simulink model "GhendyanoT2F"  (R2021b)
settings: Solver=ode45  StartTime=0.0  StopTime=TempoSimulacao  RelTol=1e-3  EnableMultiTasking=on
values from neighbouring files (symbols this model uses):
  ccc1 = Ccc*d    [TesteRealCurtoFuses.m]    (also in TesteRealCurto_SemFuse.m)
  ccc2 = Ccc*d    [TesteRealCurtoFuses.m]    (also in TesteRealCurto_SemFuse.m)
  cct1 = Cct*d    [TesteRealCurtoFuses.m]    (also in TesteRealCurto_SemFuse.m)
  cct2 = Cct*d    [TesteRealCurtoFuses.m]    (also in TesteRealCurto_SemFuse.m)
  cequa1 = Ceq*d    [TesteRealCurtoFuses.m]    (also in TesteRealCurto_SemFuse.m)
  cequa2 = Ceq*d    [TesteRealCurtoFuses.m]    (also in TesteRealCurto_SemFuse.m)
  FatorSimulacao = 1e-3    (= 0.001)    [TesteRealCurtoFuses.m]    (also in TesteRealCurto_SemFuse.m)
  le = 1e-10    [TesteRealCurto.m]    (also in TesteRealCurtoFuses.m; TesteRealCurto_SemFuse.m)
  lm1 = lm    [TesteRealCurto.m]    (also in TesteRealCurtoFuses.m; TesteRealCurto_SemFuse.m)
  lm2 = lm    [TesteRealCurto.m]    (also in TesteRealCurtoFuses.m; TesteRealCurto_SemFuse.m)
  lp1 = lp    [TesteRealCurto.m]    (also in TesteRealCurtoFuses.m; TesteRealCurto_SemFuse.m)
  lp2 = lp    [TesteRealCurto.m]    (also in TesteRealCurtoFuses.m; TesteRealCurto_SemFuse.m)
  NRE = 1e-12    [TesteRealCurto.m]    (also in TesteRealCurtoFuses.m; TesteRealCurto_SemFuse.m)
  Raf1 = inf    [TesteRealCurto.m]    (also in TesteRealCurtoFuses.m; TesteRealCurto_SemFuse.m)
  Raf2 = inf    [TesteRealCurto.m]    (also in TesteRealCurtoFuses.m; TesteRealCurto_SemFuse.m)
  Rbf1 = inf    [TesteRealCurto.m]    (also in TesteRealCurtoFuses.m; TesteRealCurto_SemFuse.m)
  Rbf2 = inf    [TesteRealCurto.m]    (also in TesteRealCurtoFuses.m; TesteRealCurto_SemFuse.m)
  Rcf1 = inf    [TesteRealCurto.m]    (also in TesteRealCurtoFuses.m; TesteRealCurto_SemFuse.m)
  Rcf2 = inf    [TesteRealCurto.m]    (also in TesteRealCurtoFuses.m; TesteRealCurto_SemFuse.m)
  rm1 = rm    [TesteRealCurto.m]    (also in TesteRealCurtoFuses.m; TesteRealCurto_SemFuse.m)
  rm2 = rm    [TesteRealCurto.m]    (also in TesteRealCurtoFuses.m; TesteRealCurto_SemFuse.m)
  rp1 = rp    [TesteRealCurto.m]    (also in TesteRealCurtoFuses.m; TesteRealCurto_SemFuse.m)
  rp2 = rp    [TesteRealCurto.m]    (also in TesteRealCurtoFuses.m; TesteRealCurto_SemFuse.m)
  rtc1 = 8    [TesteRealCurto.m]    (also in TesteRealCurtoFuses.m; TesteRealCurto_SemFuse.m)
  rtc2 = 8    [TesteRealCurto.m]    (also in TesteRealCurtoFuses.m; TesteRealCurto_SemFuse.m)
  rti = 10    [TesteRealCurto.m]    (also in TesteRealCurtoFuses.m; TesteRealCurto_SemFuse.m)
undefined symbols (not defined in the file or in its folder): D11, Delta
libraries: spsSeriesRLCBranchLib x26, spsRMSLib x14, spsBreakerLib x9, spsCurrentMeasurementLib x9, spsThreePhaseTransformerTwoWindingsLib x4, spsThreePhaseVIMeasurementLib x3, spsMutualInductanceLib x2, spsThreePhaseSeriesRLCLoadLib x2, spsThreePhaseSourceLib x1, spspowerguiLib x1
(part 1 of 2)
settings Model: Creator=laris  LastModifiedBy=Leonardo-Felipe
settings SolverCC: AlgebraicLoopSolver=TrustRegion
settings DataIOCC: LimitDataPoints=on  SaveFormat=Array  ReturnWorkspaceOutputs=off
settings OptimizationCC: LifeSpan=inf
settings DebuggingCC: SFUnexpectedBacktrackingDiag=warning  SFNoUnconditionalDefaultTransitionDiag=warning  SFExecutionAtInitializationDiag=none  SFMachineParentedDataDiag=warning  ArithmeticOperatorsInVariantConditions=warning
settings HardwareCC: ProdBitPerPointer=32  ProdBitPerSizeT=32  ProdBitPerPtrDiffT=32  ProdLargestAtomicFloat=None  ProdIntDivRoundTo=Undefined  ProdEndianess=Unspecified  ProdWordSize=32  ProdHWDeviceType=32-bit Generic
settings ModelReferenceCC: PropagateSignalLabelsOutOfModel=off
settings SFSimCC: SimUseLocalCustomCode=off  CustomCodeUndefinedFunction=UseInterfaceOnly
settings RTWCC: RTWUseLocalCustomCode=off
settings CodeAppCC: StateflowObjectComments=on
settings GRTTargetCC: TargetLangStandard=C89/C90 (ANSI)
settings ConfigComp: CovMetricSettings=dw  CovSaveCumulativeToWorkspaceVar=on  CovSaveSingleToWorkspaceVar=on  CovExternalEMLEnable=off
settings SimscapeCC: SimscapeNormalizeSystem=off

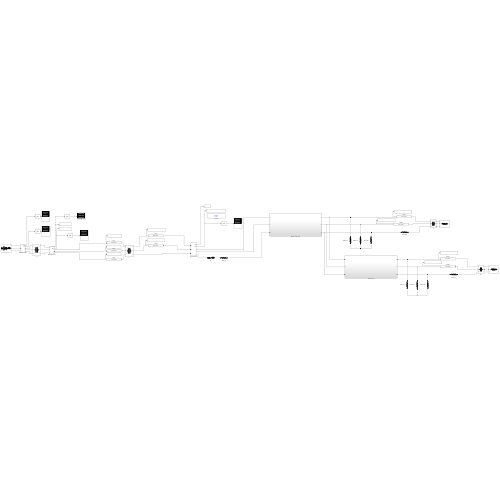
[thumbnail: Simulink's stored preview of the top-level diagram]
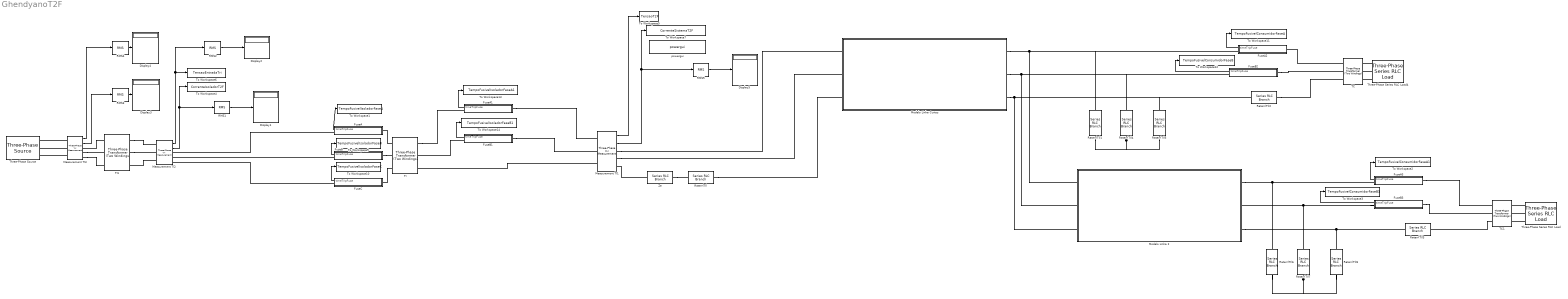
== system GhendyanoT2F ==
  Display{1..5} (5 alike) : Display
  FuseA : Subsystem  mask{tipofuse=5H, a=33.5364, b=-24.1389, c=7.0071, d=-1.0167, e=0.0569, IoTot=5}
      mask prompts: tipofuse "Tipo de Fusivel"
      mask TypeOptions tipofuse: 5H
      mask Callback tipofuse:
      | switch(get_param(gcb,'tipofuse'))
      |     case '1H'
      |         set_param(gcb,'a','11.5834');
      |         set_param(gcb,'b','-7.7159');
      |         set_param(gcb,'c','2.2435');
      |         set_param(gcb,'d','-0.4141');
      |         set_param(gcb,'e','0.0293');
      |         set_param(gcb,'IoTot','1');
      |     case '2H'
      |         set_param(gcb,'a','15.3612');
      |         set_param(gcb,'b','-11.3048');
      |         set_param(gcb,'c','3.7855');
      |         set_param(gcb,'d','-0.6767');
      |         set_param(gcb,'e','0.0442');
      |         set_param(gcb,'IoTot','2');
      |     case '3H'
      |         set_param(gcb,'a','16.6469');
      |         set_param(gcb,'b','-10.3608');
      |         set_param(gcb,'c','2.8987');
      |         set_param(gcb,'d','-0.4844');
      |         set_param(gcb,'e','0.0315');
      |         set_param(gcb,'IoTot','3');
      |     case '5H'
      |         set_param(gcb,'a','33.5364');
      |         set_param(gcb,'b','-24.1389');
      |         set_param(gcb,'c','7.0071');
      |         set_param(gcb,'d','-1.0167');
      |         set_param(gcb,'e','0.0569');
      |         set_param(gcb,'IoTot','5');
      |     case '8H'
      |         set_param(gcb,'a','137.5572');
      |         set_param(gcb,'b','-119.0117');
      |         set_param(gcb,'c','38.2794');
      |         set_param(gcb,'d','-5.4440');
      |         set_param(gcb,'e','0.2846');
      |         set_param(gcb,'IoTot','8');
      |     case '6K'
      |         set_param(gcb,'a','181.2568');
      |         set_param(gcb,'b','-167.5711');
      |         set_param(gcb,'c','57.6673');
      |         set_param(gcb,'d','-8.7672');
      |         set_param(gcb,'e','0.4916');
      |         set_param(gcb,'IoTot','6');
      |     case '8K'
      |         set_param(gcb,'a','201.6778');
      |         set_param(gcb,'b','-175.2376');
      |         set_param(gcb,'c','56.8760');
      |         set_param(gcb,'d','-8.1725');
      |         set_param(gcb,'e','0.4340');
      |         set_param(gcb,'IoTot','8');
      |     case '10K'
      |         set_param(gcb,'a','251.8801');
      |         set_param(gcb,'b','-206.6378');
      |         set_param(gcb,'c','63.3069');
      |         set_param(gcb,'d','-8.5810');
      |         set_param(gcb,'e','0.4304');
      |         set_param(gcb,'IoTot','10');
      |     case '12K'
      |         set_param(gcb,'a','294.2461');
      |         set_param(gcb,'b','-229.0340');
      |         set_param(gcb,'c','66.6693');
      |         set_param(gcb,'d','-8.5945');
      |         set_param(gcb,'e','0.4107');
      |         set_param(gcb,'IoTot','12');
      |     case '15K'
      |         set_param(gcb,'a','346.4070');
      |         set_param(gcb,'b','-257.6697');
      |         set_param(gcb,'c','71.6644');
      |         set_param(gcb,'d','-8.8225');
      |         set_param(gcb,'e','0.4027');
      |         set_param(gcb,'IoTot','15');
      |     case '20K'
      |         set_param(gcb,'a','382.4620');
      |         set_param(gcb,'b','-271.3985');
      |         set_param(gcb,'c','72.1161');
      |         set_param(gcb,'d','-8.4924');
      |         set_param(gcb,'e','0.3714');
      |         set_param(gcb,'IoTot','20');
      |     case '25K'
      |         set_param(gcb,'a','469.9755');
      |         set_param(gcb,'b','-321.2512');
      |         set_param(gcb,'c','82.1749');
      |         set_param(gcb,'d','-9.3092');
      |         set_param(gcb,'e','0.3918');
      |         set_param(gcb,'IoTot','25');
      |     case '30K'
      |         set_param(gcb,'a','516.7220');
      |         set_param(gcb,'b','-337.6034');
      |         set_param(gcb,'c','82.5876');
      |         set_param(gcb,'d','-8.9522');
      |         set_param(gcb,'e','0.3608');
      |         set_param(gcb,'IoTot','30');
      |     case '40K'
      |         set_param(gcb,'a','672.1360');
      |         set_param(gcb,'b','-424.7867');
      |         set_param(gcb,'c','100.3706');
      |         set_param(gcb,'d','-10.4950');
      |         set_param(gcb,'e','0.4080');
      |         set_param(gcb,'IoTot','40');
      |     case '50K'
      |         set_param(gcb,'a','691.3953');
      |         set_param(gcb,'b','-419.2300');
      |         set_param(gcb,'c','95.1730');
      |         set_param(gcb,'d','-9.5735');
      |         set_param(gcb,'e','0.3584');
      |         set_param(gcb,'IoTot','50');
      |     case '65K'
      |         set_param(gcb,'a','841.8993');
      |         set_param(gcb,'b','-492.8148');
      |         set_param(gcb,'c','107.9499');
      |         set_param(gcb,'d','-10.4731');
      |         set_param(gcb,'e','0.3783');
      |         set_param(gcb,'IoTot','65');
      |     case '80K'
      |         set_param(gcb,'a','881.1649');
      |         set_param(gcb,'b','-499.4578');
      |         set_param(gcb,'c','106.0005');
      |         set_param(gcb,'d','-9.9685');
      |         set_param(gcb,'e','0.3492');
      |         set_param(gcb,'IoTot','80');
      |     case '100K'
      |         set_param(gcb,'a','1020.0325');
      |         set_param(gcb,'b','-554.4466');
      |         set_param(gcb,'c','112.8674');
      |         set_param(gcb,'d','-10.1845');
      |         set_param(gcb,'e','0.3425');
      |         set_param(gcb,'IoTot','100');
      | end
      mask Display: disp('Elo Fusivel');
  FuseA1 : Subsystem  mask{tipofuse=5H, a=33.5364, b=-24.1389, c=7.0071, d=-1.0167, e=0.0569, IoTot=5}
      mask prompts: tipofuse "Tipo de Fusivel"
      mask TypeOptions tipofuse: 5H
      mask Callback tipofuse:
      | switch(get_param(gcb,'tipofuse'))
      |     case '1H'
      |         set_param(gcb,'a','11.5834');
      |         set_param(gcb,'b','-7.7159');
      |         set_param(gcb,'c','2.2435');
      |         set_param(gcb,'d','-0.4141');
      |         set_param(gcb,'e','0.0293');
      |         set_param(gcb,'IoTot','1');
      |     case '2H'
      |         set_param(gcb,'a','15.3612');
      |         set_param(gcb,'b','-11.3048');
      |         set_param(gcb,'c','3.7855');
      |         set_param(gcb,'d','-0.6767');
      |         set_param(gcb,'e','0.0442');
      |         set_param(gcb,'IoTot','2');
      |     case '3H'
      |         set_param(gcb,'a','16.6469');
      |         set_param(gcb,'b','-10.3608');
      |         set_param(gcb,'c','2.8987');
      |         set_param(gcb,'d','-0.4844');
      |         set_param(gcb,'e','0.0315');
      |         set_param(gcb,'IoTot','3');
      |     case '5H'
      |         set_param(gcb,'a','33.5364');
      |         set_param(gcb,'b','-24.1389');
      |         set_param(gcb,'c','7.0071');
      |         set_param(gcb,'d','-1.0167');
      |         set_param(gcb,'e','0.0569');
      |         set_param(gcb,'IoTot','5');
      |     case '8H'
      |         set_param(gcb,'a','137.5572');
      |         set_param(gcb,'b','-119.0117');
      |         set_param(gcb,'c','38.2794');
      |         set_param(gcb,'d','-5.4440');
      |         set_param(gcb,'e','0.2846');
      |         set_param(gcb,'IoTot','8');
      |     case '6K'
      |         set_param(gcb,'a','181.2568');
      |         set_param(gcb,'b','-167.5711');
      |         set_param(gcb,'c','57.6673');
      |         set_param(gcb,'d','-8.7672');
      |         set_param(gcb,'e','0.4916');
      |         set_param(gcb,'IoTot','6');
      |     case '8K'
      |         set_param(gcb,'a','201.6778');
      |         set_param(gcb,'b','-175.2376');
      |         set_param(gcb,'c','56.8760');
      |         set_param(gcb,'d','-8.1725');
      |         set_param(gcb,'e','0.4340');
      |         set_param(gcb,'IoTot','8');
      |     case '10K'
      |         set_param(gcb,'a','251.8801');
      |         set_param(gcb,'b','-206.6378');
      |         set_param(gcb,'c','63.3069');
      |         set_param(gcb,'d','-8.5810');
      |         set_param(gcb,'e','0.4304');
      |         set_param(gcb,'IoTot','10');
      |     case '12K'
      |         set_param(gcb,'a','294.2461');
      |         set_param(gcb,'b','-229.0340');
      |         set_param(gcb,'c','66.6693');
      |         set_param(gcb,'d','-8.5945');
      |         set_param(gcb,'e','0.4107');
      |         set_param(gcb,'IoTot','12');
      |     case '15K'
      |         set_param(gcb,'a','346.4070');
      |         set_param(gcb,'b','-257.6697');
      |         set_param(gcb,'c','71.6644');
      |         set_param(gcb,'d','-8.8225');
      |         set_param(gcb,'e','0.4027');
      |         set_param(gcb,'IoTot','15');
      |     case '20K'
      |         set_param(gcb,'a','382.4620');
      |         set_param(gcb,'b','-271.3985');
      |         set_param(gcb,'c','72.1161');
      |         set_param(gcb,'d','-8.4924');
      |         set_param(gcb,'e','0.3714');
      |         set_param(gcb,'IoTot','20');
      |     case '25K'
      |         set_param(gcb,'a','469.9755');
      |         set_param(gcb,'b','-321.2512');
      |         set_param(gcb,'c','82.1749');
      |         set_param(gcb,'d','-9.3092');
      |         set_param(gcb,'e','0.3918');
      |         set_param(gcb,'IoTot','25');
      |     case '30K'
      |         set_param(gcb,'a','516.7220');
      |         set_param(gcb,'b','-337.6034');
      |         set_param(gcb,'c','82.5876');
      |         set_param(gcb,'d','-8.9522');
      |         set_param(gcb,'e','0.3608');
      |         set_param(gcb,'IoTot','30');
      |     case '40K'
      |         set_param(gcb,'a','672.1360');
      |         set_param(gcb,'b','-424.7867');
      |         set_param(gcb,'c','100.3706');
      |         set_param(gcb,'d','-10.4950');
      |         set_param(gcb,'e','0.4080');
      |         set_param(gcb,'IoTot','40');
      |     case '50K'
      |         set_param(gcb,'a','691.3953');
      |         set_param(gcb,'b','-419.2300');
      |         set_param(gcb,'c','95.1730');
      |         set_param(gcb,'d','-9.5735');
      |         set_param(gcb,'e','0.3584');
      |         set_param(gcb,'IoTot','50');
      |     case '65K'
      |         set_param(gcb,'a','841.8993');
      |         set_param(gcb,'b','-492.8148');
      |         set_param(gcb,'c','107.9499');
      |         set_param(gcb,'d','-10.4731');
      |         set_param(gcb,'e','0.3783');
      |         set_param(gcb,'IoTot','65');
      |     case '80K'
      |         set_param(gcb,'a','881.1649');
      |         set_param(gcb,'b','-499.4578');
      |         set_param(gcb,'c','106.0005');
      |         set_param(gcb,'d','-9.9685');
      |         set_param(gcb,'e','0.3492');
      |         set_param(gcb,'IoTot','80');
      |     case '100K'
      |         set_param(gcb,'a','1020.0325');
      |         set_param(gcb,'b','-554.4466');
      |         set_param(gcb,'c','112.8674');
      |         set_param(gcb,'d','-10.1845');
      |         set_param(gcb,'e','0.3425');
      |         set_param(gcb,'IoTot','100');
      | end
      mask Display: disp('Elo Fusivel');
  FuseA2 : Subsystem  mask{tipofuse=3H, a=16.6469, b=-10.3608, c=2.8987, d=-0.4844, e=0.0315, IoTot=3}
      mask prompts: tipofuse "Tipo de Fusivel"
      mask TypeOptions tipofuse: 3H
      mask Callback tipofuse:
      | switch(get_param(gcb,'tipofuse'))
      |     case '1H'
      |         set_param(gcb,'a','11.5834');
      |         set_param(gcb,'b','-7.7159');
      |         set_param(gcb,'c','2.2435');
      |         set_param(gcb,'d','-0.4141');
      |         set_param(gcb,'e','0.0293');
      |         set_param(gcb,'IoTot','1');
      |     case '2H'
      |         set_param(gcb,'a','15.3612');
      |         set_param(gcb,'b','-11.3048');
      |         set_param(gcb,'c','3.7855');
      |         set_param(gcb,'d','-0.6767');
      |         set_param(gcb,'e','0.0442');
      |         set_param(gcb,'IoTot','2');
      |     case '3H'
      |         set_param(gcb,'a','16.6469');
      |         set_param(gcb,'b','-10.3608');
      |         set_param(gcb,'c','2.8987');
      |         set_param(gcb,'d','-0.4844');
      |         set_param(gcb,'e','0.0315');
      |         set_param(gcb,'IoTot','3');
      |     case '5H'
      |         set_param(gcb,'a','33.5364');
      |         set_param(gcb,'b','-24.1389');
      |         set_param(gcb,'c','7.0071');
      |         set_param(gcb,'d','-1.0167');
      |         set_param(gcb,'e','0.0569');
      |         set_param(gcb,'IoTot','5');
      |     case '8H'
      |         set_param(gcb,'a','137.5572');
      |         set_param(gcb,'b','-119.0117');
      |         set_param(gcb,'c','38.2794');
      |         set_param(gcb,'d','-5.4440');
      |         set_param(gcb,'e','0.2846');
      |         set_param(gcb,'IoTot','8');
      |     case '6K'
      |         set_param(gcb,'a','181.2568');
      |         set_param(gcb,'b','-167.5711');
      |         set_param(gcb,'c','57.6673');
      |         set_param(gcb,'d','-8.7672');
      |         set_param(gcb,'e','0.4916');
      |         set_param(gcb,'IoTot','6');
      |     case '8K'
      |         set_param(gcb,'a','201.6778');
      |         set_param(gcb,'b','-175.2376');
      |         set_param(gcb,'c','56.8760');
      |         set_param(gcb,'d','-8.1725');
      |         set_param(gcb,'e','0.4340');
      |         set_param(gcb,'IoTot','8');
      |     case '10K'
      |         set_param(gcb,'a','251.8801');
      |         set_param(gcb,'b','-206.6378');
      |         set_param(gcb,'c','63.3069');
      |         set_param(gcb,'d','-8.5810');
      |         set_param(gcb,'e','0.4304');
      |         set_param(gcb,'IoTot','10');
      |     case '12K'
      |         set_param(gcb,'a','294.2461');
      |         set_param(gcb,'b','-229.0340');
      |         set_param(gcb,'c','66.6693');
      |         set_param(gcb,'d','-8.5945');
      |         set_param(gcb,'e','0.4107');
      |         set_param(gcb,'IoTot','12');
      |     case '15K'
      |         set_param(gcb,'a','346.4070');
      |         set_param(gcb,'b','-257.6697');
      |         set_param(gcb,'c','71.6644');
      |         set_param(gcb,'d','-8.8225');
      |         set_param(gcb,'e','0.4027');
      |         set_param(gcb,'IoTot','15');
      |     case '20K'
      |         set_param(gcb,'a','382.4620');
      |         set_param(gcb,'b','-271.3985');
      |         set_param(gcb,'c','72.1161');
      |         set_param(gcb,'d','-8.4924');
      |         set_param(gcb,'e','0.3714');
      |         set_param(gcb,'IoTot','20');
      |     case '25K'
      |         set_param(gcb,'a','469.9755');
      |         set_param(gcb,'b','-321.2512');
      |         set_param(gcb,'c','82.1749');
      |         set_param(gcb,'d','-9.3092');
      |         set_param(gcb,'e','0.3918');
      |         set_param(gcb,'IoTot','25');
      |     case '30K'
      |         set_param(gcb,'a','516.7220');
      |         set_param(gcb,'b','-337.6034');
      |         set_param(gcb,'c','82.5876');
      |         set_param(gcb,'d','-8.9522');
      |         set_param(gcb,'e','0.3608');
      |         set_param(gcb,'IoTot','30');
      |     case '40K'
      |         set_param(gcb,'a','672.1360');
      |         set_param(gcb,'b','-424.7867');
      |         set_param(gcb,'c','100.3706');
      |         set_param(gcb,'d','-10.4950');
      |         set_param(gcb,'e','0.4080');
      |         set_param(gcb,'IoTot','40');
      |     case '50K'
      |         set_param(gcb,'a','691.3953');
      |         set_param(gcb,'b','-419.2300');
      |         set_param(gcb,'c','95.1730');
      |         set_param(gcb,'d','-9.5735');
      |         set_param(gcb,'e','0.3584');
      |         set_param(gcb,'IoTot','50');
      |     case '65K'
      |         set_param(gcb,'a','841.8993');
      |         set_param(gcb,'b','-492.8148');
      |         set_param(gcb,'c','107.9499');
      |         set_param(gcb,'d','-10.4731');
      |         set_param(gcb,'e','0.3783');
      |         set_param(gcb,'IoTot','65');
      |     case '80K'
      |         set_param(gcb,'a','881.1649');
      |         set_param(gcb,'b','-499.4578');
      |         set_param(gcb,'c','106.0005');
      |         set_param(gcb,'d','-9.9685');
      |         set_param(gcb,'e','0.3492');
      |         set_param(gcb,'IoTot','80');
      |     case '100K'
      |         set_param(gcb,'a','1020.0325');
      |         set_param(gcb,'b','-554.4466');
      |         set_param(gcb,'c','112.8674');
      |         set_param(gcb,'d','-10.1845');
      |         set_param(gcb,'e','0.3425');
      |         set_param(gcb,'IoTot','100');
      | end
      mask Display: disp('Elo Fusivel');
  FuseA3 : Subsystem  mask{tipofuse=2H, a=15.3612, b=-11.3048, c=3.7855, d=-0.6767, e=0.0442, IoTot=2}
      mask prompts: tipofuse "Tipo de Fusivel"
      mask TypeOptions tipofuse: 2H
      mask Callback tipofuse:
      | switch(get_param(gcb,'tipofuse'))
      |     case '1H'
      |         set_param(gcb,'a','11.5834');
      |         set_param(gcb,'b','-7.7159');
      |         set_param(gcb,'c','2.2435');
      |         set_param(gcb,'d','-0.4141');
      |         set_param(gcb,'e','0.0293');
      |         set_param(gcb,'IoTot','1');
      |     case '2H'
      |         set_param(gcb,'a','15.3612');
      |         set_param(gcb,'b','-11.3048');
      |         set_param(gcb,'c','3.7855');
      |         set_param(gcb,'d','-0.6767');
      |         set_param(gcb,'e','0.0442');
      |         set_param(gcb,'IoTot','2');
      |     case '3H'
      |         set_param(gcb,'a','16.6469');
      |         set_param(gcb,'b','-10.3608');
      |         set_param(gcb,'c','2.8987');
      |         set_param(gcb,'d','-0.4844');
      |         set_param(gcb,'e','0.0315');
      |         set_param(gcb,'IoTot','3');
      |     case '5H'
      |         set_param(gcb,'a','33.5364');
      |         set_param(gcb,'b','-24.1389');
      |         set_param(gcb,'c','7.0071');
      |         set_param(gcb,'d','-1.0167');
      |         set_param(gcb,'e','0.0569');
      |         set_param(gcb,'IoTot','5');
      |     case '8H'
      |         set_param(gcb,'a','137.5572');
      |         set_param(gcb,'b','-119.0117');
      |         set_param(gcb,'c','38.2794');
      |         set_param(gcb,'d','-5.4440');
      |         set_param(gcb,'e','0.2846');
      |         set_param(gcb,'IoTot','8');
      |     case '6K'
      |         set_param(gcb,'a','181.2568');
      |         set_param(gcb,'b','-167.5711');
      |         set_param(gcb,'c','57.6673');
      |         set_param(gcb,'d','-8.7672');
      |         set_param(gcb,'e','0.4916');
      |         set_param(gcb,'IoTot','6');
      |     case '8K'
      |         set_param(gcb,'a','201.6778');
      |         set_param(gcb,'b','-175.2376');
      |         set_param(gcb,'c','56.8760');
      |         set_param(gcb,'d','-8.1725');
      |         set_param(gcb,'e','0.4340');
      |         set_param(gcb,'IoTot','8');
      |     case '10K'
      |         set_param(gcb,'a','251.8801');
      |         set_param(gcb,'b','-206.6378');
      |         set_param(gcb,'c','63.3069');
      |         set_param(gcb,'d','-8.5810');
      |         set_param(gcb,'e','0.4304');
      |         set_param(gcb,'IoTot','10');
      |     case '12K'
      |         set_param(gcb,'a','294.2461');
      |         set_param(gcb,'b','-229.0340');
      |         set_param(gcb,'c','66.6693');
      |         set_param(gcb,'d','-8.5945');
      |         set_param(gcb,'e','0.4107');
      |         set_param(gcb,'IoTot','12');
      |     case '15K'
      |         set_param(gcb,'a','346.4070');
      |         set_param(gcb,'b','-257.6697');
      |         set_param(gcb,'c','71.6644');
      |         set_param(gcb,'d','-8.8225');
      |         set_param(gcb,'e','0.4027');
      |         set_param(gcb,'IoTot','15');
      |     case '20K'
      |         set_param(gcb,'a','382.4620');
      |         set_param(gcb,'b','-271.3985');
      |         set_param(gcb,'c','72.1161');
      |         set_param(gcb,'d','-8.4924');
      |         set_param(gcb,'e','0.3714');
      |         set_param(gcb,'IoTot','20');
      |     case '25K'
      |         set_param(gcb,'a','469.9755');
      |         set_param(gcb,'b','-321.2512');
      |         set_param(gcb,'c','82.1749');
      |         set_param(gcb,'d','-9.3092');
      |         set_param(gcb,'e','0.3918');
      |         set_param(gcb,'IoTot','25');
      |     case '30K'
      |         set_param(gcb,'a','516.7220');
      |         set_param(gcb,'b','-337.6034');
      |         set_param(gcb,'c','82.5876');
      |         set_param(gcb,'d','-8.9522');
      |         set_param(gcb,'e','0.3608');
      |         set_param(gcb,'IoTot','30');
      |     case '40K'
      |         set_param(gcb,'a','672.1360');
      |         set_param(gcb,'b','-424.7867');
      |         set_param(gcb,'c','100.3706');
      |         set_param(gcb,'d','-10.4950');
      |         set_param(gcb,'e','0.4080');
      |         set_param(gcb,'IoTot','40');
      |     case '50K'
      |         set_param(gcb,'a','691.3953');
      |         set_param(gcb,'b','-419.2300');
      |         set_param(gcb,'c','95.1730');
      |         set_param(gcb,'d','-9.5735');
      |         set_param(gcb,'e','0.3584');
      |         set_param(gcb,'IoTot','50');
      |     case '65K'
      |         set_param(gcb,'a','841.8993');
      |         set_param(gcb,'b','-492.8148');
      |         set_param(gcb,'c','107.9499');
      |         set_param(gcb,'d','-10.4731');
      |         set_param(gcb,'e','0.3783');
      |         set_param(gcb,'IoTot','65');
      |     case '80K'
      |         set_param(gcb,'a','881.1649');
      |         set_param(gcb,'b','-499.4578');
      |         set_param(gcb,'c','106.0005');
      |         set_param(gcb,'d','-9.9685');
      |         set_param(gcb,'e','0.3492');
      |         set_param(gcb,'IoTot','80');
      |     case '100K'
      |         set_param(gcb,'a','1020.0325');
      |         set_param(gcb,'b','-554.4466');
      |         set_param(gcb,'c','112.8674');
      |         set_param(gcb,'d','-10.1845');
      |         set_param(gcb,'e','0.3425');
      |         set_param(gcb,'IoTot','100');
      | end
      mask Display: disp('Elo Fusivel');
  FuseB : Subsystem  mask{tipofuse=5H, a=33.5364, b=-24.1389, c=7.0071, d=-1.0167, e=0.0569, IoTot=5}
      mask prompts: tipofuse "Tipo de Fusivel"
      mask TypeOptions tipofuse: 5H
      mask Callback tipofuse:
      | switch(get_param(gcb,'tipofuse'))
      |     case '1H'
      |         set_param(gcb,'a','11.5834');
      |         set_param(gcb,'b','-7.7159');
      |         set_param(gcb,'c','2.2435');
      |         set_param(gcb,'d','-0.4141');
      |         set_param(gcb,'e','0.0293');
      |         set_param(gcb,'IoTot','1');
      |     case '2H'
      |         set_param(gcb,'a','15.3612');
      |         set_param(gcb,'b','-11.3048');
      |         set_param(gcb,'c','3.7855');
      |         set_param(gcb,'d','-0.6767');
      |         set_param(gcb,'e','0.0442');
      |         set_param(gcb,'IoTot','2');
      |     case '3H'
      |         set_param(gcb,'a','16.6469');
      |         set_param(gcb,'b','-10.3608');
      |         set_param(gcb,'c','2.8987');
      |         set_param(gcb,'d','-0.4844');
      |         set_param(gcb,'e','0.0315');
      |         set_param(gcb,'IoTot','3');
      |     case '5H'
      |         set_param(gcb,'a','33.5364');
      |         set_param(gcb,'b','-24.1389');
      |         set_param(gcb,'c','7.0071');
      |         set_param(gcb,'d','-1.0167');
      |         set_param(gcb,'e','0.0569');
      |         set_param(gcb,'IoTot','5');
      |     case '8H'
      |         set_param(gcb,'a','137.5572');
      |         set_param(gcb,'b','-119.0117');
      |         set_param(gcb,'c','38.2794');
      |         set_param(gcb,'d','-5.4440');
      |         set_param(gcb,'e','0.2846');
      |         set_param(gcb,'IoTot','8');
      |     case '6K'
      |         set_param(gcb,'a','181.2568');
      |         set_param(gcb,'b','-167.5711');
      |         set_param(gcb,'c','57.6673');
      |         set_param(gcb,'d','-8.7672');
      |         set_param(gcb,'e','0.4916');
      |         set_param(gcb,'IoTot','6');
      |     case '8K'
      |         set_param(gcb,'a','201.6778');
      |         set_param(gcb,'b','-175.2376');
      |         set_param(gcb,'c','56.8760');
      |         set_param(gcb,'d','-8.1725');
      |         set_param(gcb,'e','0.4340');
      |         set_param(gcb,'IoTot','8');
      |     case '10K'
      |         set_param(gcb,'a','251.8801');
      |         set_param(gcb,'b','-206.6378');
      |         set_param(gcb,'c','63.3069');
      |         set_param(gcb,'d','-8.5810');
      |         set_param(gcb,'e','0.4304');
      |         set_param(gcb,'IoTot','10');
      |     case '12K'
      |         set_param(gcb,'a','294.2461');
      |         set_param(gcb,'b','-229.0340');
      |         set_param(gcb,'c','66.6693');
      |         set_param(gcb,'d','-8.5945');
      |         set_param(gcb,'e','0.4107');
      |         set_param(gcb,'IoTot','12');
      |     case '15K'
      |         set_param(gcb,'a','346.4070');
      |         set_param(gcb,'b','-257.6697');
      |         set_param(gcb,'c','71.6644');
      |         set_param(gcb,'d','-8.8225');
      |         set_param(gcb,'e','0.4027');
      |         set_param(gcb,'IoTot','15');
      |     case '20K'
      |         set_param(gcb,'a','382.4620');
      |         set_param(gcb,'b','-271.3985');
      |         set_param(gcb,'c','72.1161');
      |         set_param(gcb,'d','-8.4924');
      |         set_param(gcb,'e','0.3714');
      |         set_param(gcb,'IoTot','20');
      |     case '25K'
      |         set_param(gcb,'a','469.9755');
      |         set_param(gcb,'b','-321.2512');
      |         set_param(gcb,'c','82.1749');
      |         set_param(gcb,'d','-9.3092');
      |         set_param(gcb,'e','0.3918');
      |         set_param(gcb,'IoTot','25');
      |     case '30K'
      |         set_param(gcb,'a','516.7220');
      |         set_param(gcb,'b','-337.6034');
      |         set_param(gcb,'c','82.5876');
      |         set_param(gcb,'d','-8.9522');
      |         set_param(gcb,'e','0.3608');
      |         set_param(gcb,'IoTot','30');
      |     case '40K'
      |         set_param(gcb,'a','672.1360');
      |         set_param(gcb,'b','-424.7867');
      |         set_param(gcb,'c','100.3706');
      |         set_param(gcb,'d','-10.4950');
      |         set_param(gcb,'e','0.4080');
      |         set_param(gcb,'IoTot','40');
      |     case '50K'
      |         set_param(gcb,'a','691.3953');
      |         set_param(gcb,'b','-419.2300');
      |         set_param(gcb,'c','95.1730');
      |         set_param(gcb,'d','-9.5735');
      |         set_param(gcb,'e','0.3584');
      |         set_param(gcb,'IoTot','50');
      |     case '65K'
      |         set_param(gcb,'a','841.8993');
      |         set_param(gcb,'b','-492.8148');
      |         set_param(gcb,'c','107.9499');
      |         set_param(gcb,'d','-10.4731');
      |         set_param(gcb,'e','0.3783');
      |         set_param(gcb,'IoTot','65');
      |     case '80K'
      |         set_param(gcb,'a','881.1649');
      |         set_param(gcb,'b','-499.4578');
      |         set_param(gcb,'c','106.0005');
      |         set_param(gcb,'d','-9.9685');
      |         set_param(gcb,'e','0.3492');
      |         set_param(gcb,'IoTot','80');
      |     case '100K'
      |         set_param(gcb,'a','1020.0325');
      |         set_param(gcb,'b','-554.4466');
      |         set_param(gcb,'c','112.8674');
      |         set_param(gcb,'d','-10.1845');
      |         set_param(gcb,'e','0.3425');
      |         set_param(gcb,'IoTot','100');
      | end
      mask Display: disp('Elo Fusivel');
  FuseB1 : Subsystem  mask{tipofuse=5H, a=33.5364, b=-24.1389, c=7.0071, d=-1.0167, e=0.0569, IoTot=5}
      mask prompts: tipofuse "Tipo de Fusivel"
      mask TypeOptions tipofuse: 5H
      mask Callback tipofuse:
      | switch(get_param(gcb,'tipofuse'))
      |     case '1H'
      |         set_param(gcb,'a','11.5834');
      |         set_param(gcb,'b','-7.7159');
      |         set_param(gcb,'c','2.2435');
      |         set_param(gcb,'d','-0.4141');
      |         set_param(gcb,'e','0.0293');
      |         set_param(gcb,'IoTot','1');
      |     case '2H'
      |         set_param(gcb,'a','15.3612');
      |         set_param(gcb,'b','-11.3048');
      |         set_param(gcb,'c','3.7855');
      |         set_param(gcb,'d','-0.6767');
      |         set_param(gcb,'e','0.0442');
      |         set_param(gcb,'IoTot','2');
      |     case '3H'
      |         set_param(gcb,'a','16.6469');
      |         set_param(gcb,'b','-10.3608');
      |         set_param(gcb,'c','2.8987');
      |         set_param(gcb,'d','-0.4844');
      |         set_param(gcb,'e','0.0315');
      |         set_param(gcb,'IoTot','3');
      |     case '5H'
      |         set_param(gcb,'a','33.5364');
      |         set_param(gcb,'b','-24.1389');
      |         set_param(gcb,'c','7.0071');
      |         set_param(gcb,'d','-1.0167');
      |         set_param(gcb,'e','0.0569');
      |         set_param(gcb,'IoTot','5');
      |     case '8H'
      |         set_param(gcb,'a','137.5572');
      |         set_param(gcb,'b','-119.0117');
      |         set_param(gcb,'c','38.2794');
      |         set_param(gcb,'d','-5.4440');
      |         set_param(gcb,'e','0.2846');
      |         set_param(gcb,'IoTot','8');
      |     case '6K'
      |         set_param(gcb,'a','181.2568');
      |         set_param(gcb,'b','-167.5711');
      |         set_param(gcb,'c','57.6673');
      |         set_param(gcb,'d','-8.7672');
      |         set_param(gcb,'e','0.4916');
      |         set_param(gcb,'IoTot','6');
      |     case '8K'
      |         set_param(gcb,'a','201.6778');
      |         set_param(gcb,'b','-175.2376');
      |         set_param(gcb,'c','56.8760');
      |         set_param(gcb,'d','-8.1725');
      |         set_param(gcb,'e','0.4340');
      |         set_param(gcb,'IoTot','8');
      |     case '10K'
      |         set_param(gcb,'a','251.8801');
      |         set_param(gcb,'b','-206.6378');
      |         set_param(gcb,'c','63.3069');
      |         set_param(gcb,'d','-8.5810');
      |         set_param(gcb,'e','0.4304');
      |         set_param(gcb,'IoTot','10');
      |     case '12K'
      |         set_param(gcb,'a','294.2461');
      |         set_param(gcb,'b','-229.0340');
      |         set_param(gcb,'c','66.6693');
      |         set_param(gcb,'d','-8.5945');
      |         set_param(gcb,'e','0.4107');
      |         set_param(gcb,'IoTot','12');
      |     case '15K'
      |         set_param(gcb,'a','346.4070');
      |         set_param(gcb,'b','-257.6697');
      |         set_param(gcb,'c','71.6644');
      |         set_param(gcb,'d','-8.8225');
      |         set_param(gcb,'e','0.4027');
      |         set_param(gcb,'IoTot','15');
      |     case '20K'
      |         set_param(gcb,'a','382.4620');
      |         set_param(gcb,'b','-271.3985');
      |         set_param(gcb,'c','72.1161');
      |         set_param(gcb,'d','-8.4924');
      |         set_param(gcb,'e','0.3714');
      |         set_param(gcb,'IoTot','20');
      |     case '25K'
      |         set_param(gcb,'a','469.9755');
      |         set_param(gcb,'b','-321.2512');
      |         set_param(gcb,'c','82.1749');
      |         set_param(gcb,'d','-9.3092');
      |         set_param(gcb,'e','0.3918');
      |         set_param(gcb,'IoTot','25');
      |     case '30K'
      |         set_param(gcb,'a','516.7220');
      |         set_param(gcb,'b','-337.6034');
      |         set_param(gcb,'c','82.5876');
      |         set_param(gcb,'d','-8.9522');
      |         set_param(gcb,'e','0.3608');
      |         set_param(gcb,'IoTot','30');
      |     case '40K'
      |         set_param(gcb,'a','672.1360');
      |         set_param(gcb,'b','-424.7867');
      |         set_param(gcb,'c','100.3706');
      |         set_param(gcb,'d','-10.4950');
      |         set_param(gcb,'e','0.4080');
      |         set_param(gcb,'IoTot','40');
      |     case '50K'
      |         set_param(gcb,'a','691.3953');
      |         set_param(gcb,'b','-419.2300');
      |         set_param(gcb,'c','95.1730');
      |         set_param(gcb,'d','-9.5735');
      |         set_param(gcb,'e','0.3584');
      |         set_param(gcb,'IoTot','50');
      |     case '65K'
      |         set_param(gcb,'a','841.8993');
      |         set_param(gcb,'b','-492.8148');
      |         set_param(gcb,'c','107.9499');
      |         set_param(gcb,'d','-10.4731');
      |         set_param(gcb,'e','0.3783');
      |         set_param(gcb,'IoTot','65');
      |     case '80K'
      |         set_param(gcb,'a','881.1649');
      |         set_param(gcb,'b','-499.4578');
      |         set_param(gcb,'c','106.0005');
      |         set_param(gcb,'d','-9.9685');
      |         set_param(gcb,'e','0.3492');
      |         set_param(gcb,'IoTot','80');
      |     case '100K'
      |         set_param(gcb,'a','1020.0325');
      |         set_param(gcb,'b','-554.4466');
      |         set_param(gcb,'c','112.8674');
      |         set_param(gcb,'d','-10.1845');
      |         set_param(gcb,'e','0.3425');
      |         set_param(gcb,'IoTot','100');
      | end
      mask Display: disp('Elo Fusivel');
  FuseB2 : Subsystem  mask{tipofuse=3H, a=16.6469, b=-10.3608, c=2.8987, d=-0.4844, e=0.0315, IoTot=3}
      mask prompts: tipofuse "Tipo de Fusivel"
      mask TypeOptions tipofuse: 3H
      mask Callback tipofuse:
      | switch(get_param(gcb,'tipofuse'))
      |     case '1H'
      |         set_param(gcb,'a','11.5834');
      |         set_param(gcb,'b','-7.7159');
      |         set_param(gcb,'c','2.2435');
      |         set_param(gcb,'d','-0.4141');
      |         set_param(gcb,'e','0.0293');
      |         set_param(gcb,'IoTot','1');
      |     case '2H'
      |         set_param(gcb,'a','15.3612');
      |         set_param(gcb,'b','-11.3048');
      |         set_param(gcb,'c','3.7855');
      |         set_param(gcb,'d','-0.6767');
      |         set_param(gcb,'e','0.0442');
      |         set_param(gcb,'IoTot','2');
      |     case '3H'
      |         set_param(gcb,'a','16.6469');
      |         set_param(gcb,'b','-10.3608');
      |         set_param(gcb,'c','2.8987');
      |         set_param(gcb,'d','-0.4844');
      |         set_param(gcb,'e','0.0315');
      |         set_param(gcb,'IoTot','3');
      |     case '5H'
      |         set_param(gcb,'a','33.5364');
      |         set_param(gcb,'b','-24.1389');
      |         set_param(gcb,'c','7.0071');
      |         set_param(gcb,'d','-1.0167');
      |         set_param(gcb,'e','0.0569');
      |         set_param(gcb,'IoTot','5');
      |     case '8H'
      |         set_param(gcb,'a','137.5572');
      |         set_param(gcb,'b','-119.0117');
      |         set_param(gcb,'c','38.2794');
      |         set_param(gcb,'d','-5.4440');
      |         set_param(gcb,'e','0.2846');
      |         set_param(gcb,'IoTot','8');
      |     case '6K'
      |         set_param(gcb,'a','181.2568');
      |         set_param(gcb,'b','-167.5711');
      |         set_param(gcb,'c','57.6673');
      |         set_param(gcb,'d','-8.7672');
      |         set_param(gcb,'e','0.4916');
      |         set_param(gcb,'IoTot','6');
      |     case '8K'
      |         set_param(gcb,'a','201.6778');
      |         set_param(gcb,'b','-175.2376');
      |         set_param(gcb,'c','56.8760');
      |         set_param(gcb,'d','-8.1725');
      |         set_param(gcb,'e','0.4340');
      |         set_param(gcb,'IoTot','8');
      |     case '10K'
      |         set_param(gcb,'a','251.8801');
      |         set_param(gcb,'b','-206.6378');
      |         set_param(gcb,'c','63.3069');
      |         set_param(gcb,'d','-8.5810');
      |         set_param(gcb,'e','0.4304');
      |         set_param(gcb,'IoTot','10');
      |     case '12K'
      |         set_param(gcb,'a','294.2461');
      |         set_param(gcb,'b','-229.0340');
      |         set_param(gcb,'c','66.6693');
      |         set_param(gcb,'d','-8.5945');
      |         set_param(gcb,'e','0.4107');
      |         set_param(gcb,'IoTot','12');
      |     case '15K'
      |         set_param(gcb,'a','346.4070');
      |         set_param(gcb,'b','-257.6697');
      |         set_param(gcb,'c','71.6644');
      |         set_param(gcb,'d','-8.8225');
      |         set_param(gcb,'e','0.4027');
      |         set_param(gcb,'IoTot','15');
      |     case '20K'
      |         set_param(gcb,'a','382.4620');
      |         set_param(gcb,'b','-271.3985');
      |         set_param(gcb,'c','72.1161');
      |         set_param(gcb,'d','-8.4924');
      |         set_param(gcb,'e','0.3714');
      |         set_param(gcb,'IoTot','20');
      |     case '25K'
      |         set_param(gcb,'a','469.9755');
      |         set_param(gcb,'b','-321.2512');
      |         set_param(gcb,'c','82.1749');
      |         set_param(gcb,'d','-9.3092');
      |         set_param(gcb,'e','0.3918');
      |         set_param(gcb,'IoTot','25');
      |     case '30K'
      |         set_param(gcb,'a','516.7220');
      |         set_param(gcb,'b','-337.6034');
      |         set_param(gcb,'c','82.5876');
      |         set_param(gcb,'d','-8.9522');
      |         set_param(gcb,'e','0.3608');
      |         set_param(gcb,'IoTot','30');
      |     case '40K'
      |         set_param(gcb,'a','672.1360');
      |         set_param(gcb,'b','-424.7867');
      |         set_param(gcb,'c','100.3706');
      |         set_param(gcb,'d','-10.4950');
      |         set_param(gcb,'e','0.4080');
      |         set_param(gcb,'IoTot','40');
      |     case '50K'
      |         set_param(gcb,'a','691.3953');
      |         set_param(gcb,'b','-419.2300');
      |         set_param(gcb,'c','95.1730');
      |         set_param(gcb,'d','-9.5735');
      |         set_param(gcb,'e','0.3584');
      |         set_param(gcb,'IoTot','50');
      |     case '65K'
      |         set_param(gcb,'a','841.8993');
      |         set_param(gcb,'b','-492.8148');
      |         set_param(gcb,'c','107.9499');
      |         set_param(gcb,'d','-10.4731');
      |         set_param(gcb,'e','0.3783');
      |         set_param(gcb,'IoTot','65');
      |     case '80K'
      |         set_param(gcb,'a','881.1649');
      |         set_param(gcb,'b','-499.4578');
      |         set_param(gcb,'c','106.0005');
      |         set_param(gcb,'d','-9.9685');
      |         set_param(gcb,'e','0.3492');
      |         set_param(gcb,'IoTot','80');
      |     case '100K'
      |         set_param(gcb,'a','1020.0325');
      |         set_param(gcb,'b','-554.4466');
      |         set_param(gcb,'c','112.8674');
      |         set_param(gcb,'d','-10.1845');
      |         set_param(gcb,'e','0.3425');
      |         set_param(gcb,'IoTot','100');
      | end
      mask Display: disp('Elo Fusivel');
  FuseB3 : Subsystem  mask{tipofuse=2H, a=15.3612, b=-11.3048, c=3.7855, d=-0.6767, e=0.0442, IoTot=2}
      mask prompts: tipofuse "Tipo de Fusivel"
      mask TypeOptions tipofuse: 2H
      mask Callback tipofuse:
      | switch(get_param(gcb,'tipofuse'))
      |     case '1H'
      |         set_param(gcb,'a','11.5834');
      |         set_param(gcb,'b','-7.7159');
      |         set_param(gcb,'c','2.2435');
      |         set_param(gcb,'d','-0.4141');
      |         set_param(gcb,'e','0.0293');
      |         set_param(gcb,'IoTot','1');
      |     case '2H'
      |         set_param(gcb,'a','15.3612');
      |         set_param(gcb,'b','-11.3048');
      |         set_param(gcb,'c','3.7855');
      |         set_param(gcb,'d','-0.6767');
      |         set_param(gcb,'e','0.0442');
      |         set_param(gcb,'IoTot','2');
      |     case '3H'
      |         set_param(gcb,'a','16.6469');
      |         set_param(gcb,'b','-10.3608');
      |         set_param(gcb,'c','2.8987');
      |         set_param(gcb,'d','-0.4844');
      |         set_param(gcb,'e','0.0315');
      |         set_param(gcb,'IoTot','3');
      |     case '5H'
      |         set_param(gcb,'a','33.5364');
      |         set_param(gcb,'b','-24.1389');
      |         set_param(gcb,'c','7.0071');
      |         set_param(gcb,'d','-1.0167');
      |         set_param(gcb,'e','0.0569');
      |         set_param(gcb,'IoTot','5');
      |     case '8H'
      |         set_param(gcb,'a','137.5572');
      |         set_param(gcb,'b','-119.0117');
      |         set_param(gcb,'c','38.2794');
      |         set_param(gcb,'d','-5.4440');
      |         set_param(gcb,'e','0.2846');
      |         set_param(gcb,'IoTot','8');
      |     case '6K'
      |         set_param(gcb,'a','181.2568');
      |         set_param(gcb,'b','-167.5711');
      |         set_param(gcb,'c','57.6673');
      |         set_param(gcb,'d','-8.7672');
      |         set_param(gcb,'e','0.4916');
      |         set_param(gcb,'IoTot','6');
      |     case '8K'
      |         set_param(gcb,'a','201.6778');
      |         set_param(gcb,'b','-175.2376');
      |         set_param(gcb,'c','56.8760');
      |         set_param(gcb,'d','-8.1725');
      |         set_param(gcb,'e','0.4340');
      |         set_param(gcb,'IoTot','8');
      |     case '10K'
      |         set_param(gcb,'a','251.8801');
      |         set_param(gcb,'b','-206.6378');
      |         set_param(gcb,'c','63.3069');
      |         set_param(gcb,'d','-8.5810');
      |         set_param(gcb,'e','0.4304');
      |         set_param(gcb,'IoTot','10');
      |     case '12K'
      |         set_param(gcb,'a','294.2461');
      |         set_param(gcb,'b','-229.0340');
      |         set_param(gcb,'c','66.6693');
      |         set_param(gcb,'d','-8.5945');
      |         set_param(gcb,'e','0.4107');
      |         set_param(gcb,'IoTot','12');
      |     case '15K'
      |         set_param(gcb,'a','346.4070');
      |         set_param(gcb,'b','-257.6697');
      |         set_param(gcb,'c','71.6644');
      |         set_param(gcb,'d','-8.8225');
      |         set_param(gcb,'e','0.4027');
      |         set_param(gcb,'IoTot','15');
      |     case '20K'
      |         set_param(gcb,'a','382.4620');
      |         set_param(gcb,'b','-271.3985');
      |         set_param(gcb,'c','72.1161');
      |         set_param(gcb,'d','-8.4924');
      |         set_param(gcb,'e','0.3714');
      |         set_param(gcb,'IoTot','20');
      |     case '25K'
      |         set_param(gcb,'a','469.9755');
      |         set_param(gcb,'b','-321.2512');
      |         set_param(gcb,'c','82.1749');
      |         set_param(gcb,'d','-9.3092');
      |         set_param(gcb,'e','0.3918');
      |         set_param(gcb,'IoTot','25');
      |     case '30K'
      |         set_param(gcb,'a','516.7220');
      |         set_param(gcb,'b','-337.6034');
      |         set_param(gcb,'c','82.5876');
      |         set_param(gcb,'d','-8.9522');
      |         set_param(gcb,'e','0.3608');
      |         set_param(gcb,'IoTot','30');
      |     case '40K'
      |         set_param(gcb,'a','672.1360');
      |         set_param(gcb,'b','-424.7867');
      |         set_param(gcb,'c','100.3706');
      |         set_param(gcb,'d','-10.4950');
      |         set_param(gcb,'e','0.4080');
      |         set_param(gcb,'IoTot','40');
      |     case '50K'
      |         set_param(gcb,'a','691.3953');
      |         set_param(gcb,'b','-419.2300');
      |         set_param(gcb,'c','95.1730');
      |         set_param(gcb,'d','-9.5735');
      |         set_param(gcb,'e','0.3584');
      |         set_param(gcb,'IoTot','50');
      |     case '65K'
      |         set_param(gcb,'a','841.8993');
      |         set_param(gcb,'b','-492.8148');
      |         set_param(gcb,'c','107.9499');
      |         set_param(gcb,'d','-10.4731');
      |         set_param(gcb,'e','0.3783');
      |         set_param(gcb,'IoTot','65');
      |     case '80K'
      |         set_param(gcb,'a','881.1649');
      |         set_param(gcb,'b','-499.4578');
      |         set_param(gcb,'c','106.0005');
      |         set_param(gcb,'d','-9.9685');
      |         set_param(gcb,'e','0.3492');
      |         set_param(gcb,'IoTot','80');
      |     case '100K'
      |         set_param(gcb,'a','1020.0325');
      |         set_param(gcb,'b','-554.4466');
      |         set_param(gcb,'c','112.8674');
      |         set_param(gcb,'d','-10.1845');
      |         set_param(gcb,'e','0.3425');
      |         set_param(gcb,'IoTot','100');
      | end
      mask Display: disp('Elo Fusivel');
  FuseC : Subsystem  mask{tipofuse=5H, a=33.5364, b=-24.1389, c=7.0071, d=-1.0167, e=0.0569, IoTot=5}
      mask prompts: tipofuse "Tipo de Fusivel"
      mask TypeOptions tipofuse: 5H
      mask Callback tipofuse:
      | switch(get_param(gcb,'tipofuse'))
      |     case '1H'
      |         set_param(gcb,'a','11.5834');
      |         set_param(gcb,'b','-7.7159');
      |         set_param(gcb,'c','2.2435');
      |         set_param(gcb,'d','-0.4141');
      |         set_param(gcb,'e','0.0293');
      |         set_param(gcb,'IoTot','1');
      |     case '2H'
      |         set_param(gcb,'a','15.3612');
      |         set_param(gcb,'b','-11.3048');
      |         set_param(gcb,'c','3.7855');
      |         set_param(gcb,'d','-0.6767');
      |         set_param(gcb,'e','0.0442');
      |         set_param(gcb,'IoTot','2');
      |     case '3H'
      |         set_param(gcb,'a','16.6469');
      |         set_param(gcb,'b','-10.3608');
      |         set_param(gcb,'c','2.8987');
      |         set_param(gcb,'d','-0.4844');
      |         set_param(gcb,'e','0.0315');
      |         set_param(gcb,'IoTot','3');
      |     case '5H'
      |         set_param(gcb,'a','33.5364');
      |         set_param(gcb,'b','-24.1389');
      |         set_param(gcb,'c','7.0071');
      |         set_param(gcb,'d','-1.0167');
      |         set_param(gcb,'e','0.0569');
      |         set_param(gcb,'IoTot','5');
      |     case '8H'
      |         set_param(gcb,'a','137.5572');
      |         set_param(gcb,'b','-119.0117');
      |         set_param(gcb,'c','38.2794');
      |         set_param(gcb,'d','-5.4440');
      |         set_param(gcb,'e','0.2846');
      |         set_param(gcb,'IoTot','8');
      |     case '6K'
      |         set_param(gcb,'a','181.2568');
      |         set_param(gcb,'b','-167.5711');
      |         set_param(gcb,'c','57.6673');
      |         set_param(gcb,'d','-8.7672');
      |         set_param(gcb,'e','0.4916');
      |         set_param(gcb,'IoTot','6');
      |     case '8K'
      |         set_param(gcb,'a','201.6778');
      |         set_param(gcb,'b','-175.2376');
      |         set_param(gcb,'c','56.8760');
      |         set_param(gcb,'d','-8.1725');
      |         set_param(gcb,'e','0.4340');
      |         set_param(gcb,'IoTot','8');
      |     case '10K'
      |         set_param(gcb,'a','251.8801');
      |         set_param(gcb,'b','-206.6378');
      |         set_param(gcb,'c','63.3069');
      |         set_param(gcb,'d','-8.5810');
      |         set_param(gcb,'e','0.4304');
      |         set_param(gcb,'IoTot','10');
      |     case '12K'
      |         set_param(gcb,'a','294.2461');
      |         set_param(gcb,'b','-229.0340');
      |         set_param(gcb,'c','66.6693');
      |         set_param(gcb,'d','-8.5945');
      |         set_param(gcb,'e','0.4107');
      |         set_param(gcb,'IoTot','12');
      |     case '15K'
      |         set_param(gcb,'a','346.4070');
      |         set_param(gcb,'b','-257.6697');
      |         set_param(gcb,'c','71.6644');
      |         set_param(gcb,'d','-8.8225');
      |         set_param(gcb,'e','0.4027');
      |         set_param(gcb,'IoTot','15');
      |     case '20K'
      |         set_param(gcb,'a','382.4620');
      |         set_param(gcb,'b','-271.3985');
      |         set_param(gcb,'c','72.1161');
      |         set_param(gcb,'d','-8.4924');
      |         set_param(gcb,'e','0.3714');
      |         set_param(gcb,'IoTot','20');
      |     case '25K'
      |         set_param(gcb,'a','469.9755');
      |         set_param(gcb,'b','-321.2512');
      |         set_param(gcb,'c','82.1749');
      |         set_param(gcb,'d','-9.3092');
      |         set_param(gcb,'e','0.3918');
      |         set_param(gcb,'IoTot','25');
      |     case '30K'
      |         set_param(gcb,'a','516.7220');
      |         set_param(gcb,'b','-337.6034');
      |         set_param(gcb,'c','82.5876');
      |         set_param(gcb,'d','-8.9522');
      |         set_param(gcb,'e','0.3608');
      |         set_param(gcb,'IoTot','30');
      |     case '40K'
      |         set_param(gcb,'a','672.1360');
      |         set_param(gcb,'b','-424.7867');
      |         set_param(gcb,'c','100.3706');
      |         set_param(gcb,'d','-10.4950');
      |         set_param(gcb,'e','0.4080');
      |         set_param(gcb,'IoTot','40');
      |     case '50K'
      |         set_param(gcb,'a','691.3953');
      |         set_param(gcb,'b','-419.2300');
      |         set_param(gcb,'c','95.1730');
      |         set_param(gcb,'d','-9.5735');
      |         set_param(gcb,'e','0.3584');
      |         set_param(gcb,'IoTot','50');
      |     case '65K'
      |         set_param(gcb,'a','841.8993');
      |         set_param(gcb,'b','-492.8148');
      |         set_param(gcb,'c','107.9499');
      |         set_param(gcb,'d','-10.4731');
      |         set_param(gcb,'e','0.3783');
      |         set_param(gcb,'IoTot','65');
      |     case '80K'
      |         set_param(gcb,'a','881.1649');
      |         set_param(gcb,'b','-499.4578');
      |         set_param(gcb,'c','106.0005');
      |         set_param(gcb,'d','-9.9685');
      |         set_param(gcb,'e','0.3492');
      |         set_param(gcb,'IoTot','80');
      |     case '100K'
      |         set_param(gcb,'a','1020.0325');
      |         set_param(gcb,'b','-554.4466');
      |         set_param(gcb,'c','112.8674');
      |         set_param(gcb,'d','-10.1845');
      |         set_param(gcb,'e','0.3425');
      |         set_param(gcb,'IoTot','100');
      | end
      mask Display: disp('Elo Fusivel');
  Measurement TI1 : spsThreePhaseVIMeasurementLib/Three-Phase V-I Measurement  VoltageMeasurement=phase-to-phase  SetLabelV=off  LabelV=Vabc  Vpu=off  VpuLL=off  CurrentMeasurement=yes  SetLabelI=off  LabelI=Iabc  Ipu=off  Pbase=100e6  Vbase=500e3  OutputType=Complex  PhasorSimulation=off  PSBequivalent=0
  Measurement TI2 : spsThreePhaseVIMeasurementLib/Three-Phase V-I Measurement  VoltageMeasurement=phase-to-phase  SetLabelV=off  LabelV=Vabc  Vpu=off  VpuLL=off  CurrentMeasurement=yes  SetLabelI=off  LabelI=Iabc  Ipu=off  Pbase=100e6  Vbase=500e3  OutputType=Complex  PhasorSimulation=off  PSBequivalent=0
  Measurement TI3 : spsThreePhaseVIMeasurementLib/Three-Phase V-I Measurement  VoltageMeasurement=phase-to-phase  SetLabelV=off  LabelV=Vabc  Vpu=off  VpuLL=off  CurrentMeasurement=yes  SetLabelI=off  LabelI=Iabc  Ipu=off  Pbase=100e6  Vbase=500e3  OutputType=Complex  PhasorSimulation=off  PSBequivalent=0
  Modelo Linha 2 : Subsystem
  Modelo Linha Curtos : Subsystem
  RMS{1..5} (5 alike) : spsRMSLib/RMS  TrueRMS=on  Freq=60  RMSInit=120  Ts=0
  Raterr(TI) : spsSeriesRLCBranchLib/Series RLC Branch  LConnTagsString=__new0  RConnTagsString=__new0  BranchType=R  Resistance=rti  Inductance=0  SetiL0=off  InitialCurrent=0  Capacitance=1e-6  Setx0=off  InitialVoltage=0  Measurements=None
  Raterr(TI)1 : spsSeriesRLCBranchLib/Series RLC Branch  LConnTagsString=__new0  RConnTagsString=__new0  BranchType=R  Resistance=Raf1  Inductance=0  SetiL0=off  InitialCurrent=0  Capacitance=1e-6  Setx0=off  InitialVoltage=0  Measurements=None
  Raterr(TI)2 : spsSeriesRLCBranchLib/Series RLC Branch  LConnTagsString=__new0  RConnTagsString=__new0  BranchType=R  Resistance=rtc1  Inductance=0  SetiL0=off  InitialCurrent=0  Capacitance=1e-6  Setx0=off  InitialVoltage=0  Measurements=None
  Raterr(TI)3 : spsSeriesRLCBranchLib/Series RLC Branch  LConnTagsString=__new0  RConnTagsString=__new0  BranchType=R  Resistance=rtc2  Inductance=0  SetiL0=off  InitialCurrent=0  Capacitance=1e-6  Setx0=off  InitialVoltage=0  Measurements=None
  Raterr(TI)4 : spsSeriesRLCBranchLib/Series RLC Branch  LConnTagsString=__new0  RConnTagsString=__new0  BranchType=R  Resistance=Rbf1  Inductance=0  SetiL0=off  InitialCurrent=0  Capacitance=1e-6  Setx0=off  InitialVoltage=0  Measurements=None
  Raterr(TI)5 : spsSeriesRLCBranchLib/Series RLC Branch  LConnTagsString=__new0  RConnTagsString=__new0  BranchType=R  Resistance=Rcf1  Inductance=0  SetiL0=off  InitialCurrent=0  Capacitance=1e-6  Setx0=off  InitialVoltage=0  Measurements=None
  Raterr(TI)6 : spsSeriesRLCBranchLib/Series RLC Branch  LConnTagsString=__new0  RConnTagsString=__new0  BranchType=R  Resistance=Raf2  Inductance=0  SetiL0=off  InitialCurrent=0  Capacitance=1e-6  Setx0=off  InitialVoltage=0  Measurements=None
  Raterr(TI)7 : spsSeriesRLCBranchLib/Series RLC Branch  LConnTagsString=__new0  RConnTagsString=__new0  BranchType=R  Resistance=Rbf2  Inductance=0  SetiL0=off  InitialCurrent=0  Capacitance=1e-6  Setx0=off  InitialVoltage=0  Measurements=None
  Raterr(TI)8 : spsSeriesRLCBranchLib/Series RLC Branch  LConnTagsString=__new0  RConnTagsString=__new0  BranchType=R  Resistance=Rcf2  Inductance=0  SetiL0=off  InitialCurrent=0  Capacitance=1e-6  Setx0=off  InitialVoltage=0  Measurements=None
  TC : spsThreePhaseTransformerTwoWindingsLib/Three-Phase Transformer (Two Windings)  Winding1Connection=Delta (D11)  Winding2Connection=Yg  CoreType=Three single-phase transformers  SetSaturation=off  Hysteresis=off  DataFile='hysteresis'  SetInitialFlux=off  Measurements=None  UNITS=pu  NominalPower=[75e3 , 60]  Winding1=[13800 0.0048118 0.018511]  Winding2=[380 0.0048119 0.018511]  Rm=5.801193266567229e+02*1000  Lm=8.409977380031759e+02*1000  L0=0.50001  Saturation=[0 0;0.0012545 0.01913;0.52272 0.024231]  InitialFluxes=[0.66025 -0.66025 0.57767]  BreakLoop=off  DiscreteSolver=Trapezoidal iterative  DataType=off  TransfoNumber=1
  TC1 : spsThreePhaseTransformerTwoWindingsLib/Three-Phase Transformer (Two Windings)  Winding1Connection=Delta (D11)  Winding2Connection=Yg  CoreType=Three single-phase transformers  SetSaturation=off  Hysteresis=off  DataFile='hysteresis'  SetInitialFlux=off  Measurements=None  UNITS=pu  NominalPower=[45e3 , 60]  Winding1=[13800 0.0048118 0.018511]  Winding2=[380 0.0048119 0.018511]  Rm=5.801193266567229e+02*1000  Lm=8.409977380031759e+02*1000  L0=0.50001  Saturation=[0 0;0.0012545 0.01913;0.52272 0.024231]  InitialFluxes=[0.66025 -0.66025 0.57767]  BreakLoop=off  DiscreteSolver=Trapezoidal iterative  DataType=off  TransfoNumber=1
  TI : spsThreePhaseTransformerTwoWindingsLib/Three-Phase Transformer (Two Windings)  Winding1Connection=Delta (D11)  Winding2Connection=Y  CoreType=Three single-phase transformers  SetSaturation=off  Hysteresis=off  DataFile='hysteresis'  SetInitialFlux=off  Measurements=None  UNITS=pu  NominalPower=[75e3 , 60 ]  Winding1=[13800 0.0048119 0.018511]  Winding2=[13800 0.0048119 0.018511]  Rm=1.730769230769231e+03*1000  Lm=40.010686750359440*1000  L0=6.3145  Saturation=[0 0;0.0012545 0.01913;0.52272 0.024231]  InitialFluxes=[34.179 -34.179 29.906]  BreakLoop=off  DiscreteSolver=Trapezoidal iterative  DataType=off  TransfoNumber=1
  TI1 : spsThreePhaseTransformerTwoWindingsLib/Three-Phase Transformer (Two Windings)  Winding1Connection=Yg  Winding2Connection=Delta (D11)  CoreType=Three single-phase transformers  SetSaturation=off  Hysteresis=off  DataFile='hysteresis'  SetInitialFlux=off  Measurements=None  UNITS=pu  NominalPower=[75e3 , 60 ]  Winding1=[380 0.0048119 0.018511]  Winding2=[13800 0.0048119 0.018511]  Rm=1.730769230769231e+03*1000  Lm=40.010686750359440*1000  L0=6.3145  Saturation=[0 0;0.0012545 0.01913;0.52272 0.024231]  InitialFluxes=[34.179 -34.179 29.906]  BreakLoop=off  DiscreteSolver=Trapezoidal iterative  DataType=off  TransfoNumber=1
  Three-Phase Series RLC Load : spsThreePhaseSeriesRLCLoadLib/Three-Phase Series RLC Load  LConnTagsString=A|B|C  Configuration=Y (grounded)  NominalVoltage=380  Vabc=[1e3 1e3 1e3]  Vabcp=[1e3 1e3 1e3]  NominalFrequency=60  UnbalancedPower=off  ActivePower=45e3  InductivePower=0  CapacitivePower=0  Pabc=[10e3 9e3 11e3]  QLabc=[100 90 110]  QCabc=[100 90 110]  Pabcp=[10e3 9e3 11e3]  QLabcp=[100 90 110]  QCabcp=[100 90 110]  Measurements=None  LoadType=constant Z
  Three-Phase Series RLC Load4 : spsThreePhaseSeriesRLCLoadLib/Three-Phase Series RLC Load  LConnTagsString=A|B|C  Configuration=Y (grounded)  NominalVoltage=380  Vabc=[1e3 1e3 1e3]  Vabcp=[1e3 1e3 1e3]  NominalFrequency=60  UnbalancedPower=off  ActivePower=75e3  InductivePower=0  CapacitivePower=0  Pabc=[10e3 9e3 11e3]  QLabc=[100 90 110]  QCabc=[100 90 110]  Pabcp=[10e3 9e3 11e3]  QLabcp=[100 90 110]  QCabcp=[100 90 110]  Measurements=None  LoadType=constant Z
  Three-Phase Source : spsThreePhaseSourceLib/Three-Phase Source  InternalConnection=Yg  VoltagePhases=off  Voltage=380  PhaseAngle=0  Voltage_phases=[25e3 25e3 25e3]/sqrt(3)  PhaseAngles_phases=[0 -120 +120]  Frequency=60  NonIdealSource=on  SpecifyImpedance=on  Resistance=0.8929  Inductance=16.58e-3  ShortCircuitLevel=120e6  BaseVoltage=380  XRratio=7  BusType=swing  Pref=10e3  Qref=0  Prefabc=[10e3, 10e3, 10e3]  Qrefabc=[0, 0, 0]  Qmin=-inf  Qmax=inf
  To Workspace1 : ToWorkspace  VariableName=TempoFusivelIsoladorFaseA  SampleTime=-1
      settings: MaxDataPoints=1  Save2DSignal=2-D array (concatenate along first dimension)
  To Workspace10 : ToWorkspace  VariableName=TempoFusivelIsoladorFaseC  SampleTime=-1
      settings: MaxDataPoints=1  Save2DSignal=2-D array (concatenate along first dimension)
  To Workspace11 : ToWorkspace  VariableName=TempoFusivelConsumidorFaseA  SampleTime=-1
      settings: MaxDataPoints=1  Save2DSignal=2-D array (concatenate along first dimension)
  To Workspace12 : ToWorkspace  VariableName=TempoFusivelConsumidorFaseB  SampleTime=-1
      settings: MaxDataPoints=1  Save2DSignal=2-D array (concatenate along first dimension)
  To Workspace13 : ToWorkspace  VariableName=TempoFusivelIsoladorFaseA1  SampleTime=-1
      settings: MaxDataPoints=1  Save2DSignal=2-D array (concatenate along first dimension)
  To Workspace14 : ToWorkspace  VariableName=TempoFusivelIsoladorFaseB1  SampleTime=-1
      settings: MaxDataPoints=1  Save2DSignal=2-D array (concatenate along first dimension)
  To Workspace2 : ToWorkspace  VariableName=TempoFusivelConsumidorFaseA1  SampleTime=-1
      settings: MaxDataPoints=1  Save2DSignal=2-D array (concatenate along first dimension)
  To Workspace3 : ToWorkspace  VariableName=TempoFusivelConsumidorFaseB1  SampleTime=-1
      settings: MaxDataPoints=1  Save2DSignal=2-D array (concatenate along first dimension)
  To Workspace4 : ToWorkspace  VariableName=CorrenteIsoladorT2F  SampleTime=-1
      settings: MaxDataPoints=1
  To Workspace5 : ToWorkspace  VariableName=TensaoT2F  SampleTime=-1
      settings: MaxDataPoints=1
  To Workspace6 : ToWorkspace  VariableName=TensaoEntradaTri  SampleTime=-1
      settings: MaxDataPoints=1
  To Workspace7 : ToWorkspace  VariableName=CorrenteSistemaT2F  SampleTime=-1
      settings: MaxDataPoints=1
  To Workspace9 : ToWorkspace  VariableName=TempoFusivelIsoladorFaseB  SampleTime=-1
      settings: MaxDataPoints=1  Save2DSignal=2-D array (concatenate along first dimension)
  Ze : spsSeriesRLCBranchLib/Series RLC Branch  LConnTagsString=__new0  RConnTagsString=__new0  BranchType=RL  Resistance=NRE  Inductance=le  SetiL0=off  InitialCurrent=0  Capacitance=le  Setx0=off  InitialVoltage=0  Measurements=None
  powergui : spspowerguiLib/powergui  Priority=1  SimulationMode=Discrete  SampleTime=FatorSimulacao  frequency=60  Iterations=50  frequencyindice=60  Pbase=100e6  ErrMax=1e-4  UnitsV=kV  UnitsW=MW  buscounter=0  FunctionMessages=off  echomessages=off  EnableUseOfTLC=off  CurrentSourceSwitches=off  DisableSnubberDevices=off  DisableRonSwitches=off  DisableVfSwitches=off  DisplayEquations=off  AutomaticDiscreteSolvers=off  SolverType=Tustin/Backward Euler (TBE)  Interpol=off  ExternalGateDelay=off  methode=off  Ts=100  x0status=blocks  SPID=on  SwTol=0  HookPort=off  NonlinearTolerance=1e-4  nMaxIteration=100  ContinueOnMaxIteration=off  RestoreLinks=warning  ResistiveCurrentMeasurement=off  Frange=[0:2:500]  Ylog=off  Xlog=on  ShowGrid=off  save=off  variable=ZData  structure=0  ZoomFFT=off  StartTime=0.0  cycles=1  DisplayStyle=1  fundamental=60  FreqAxis=off  MaxFrequency=1000  frequencyindicesteady=1  RmsSteady=1  display=off
  wires:
  Measurement TI1/1 -> To Workspace5/1
  FuseB/1(timeTripFuse) -> To Workspace9/1
  FuseC/1(timeTripFuse) -> To Workspace10/1
  FuseA/1(timeTripFuse) -> To Workspace1/1
  FuseB1/1(timeTripFuse) -> To Workspace14/1
  FuseA1/1(timeTripFuse) -> To Workspace13/1
  FuseA2/1(timeTripFuse) -> To Workspace11/1
  FuseB2/1(timeTripFuse) -> To Workspace12/1
  FuseB3/1(timeTripFuse) -> To Workspace3/1
  FuseA3/1(timeTripFuse) -> To Workspace2/1
  Measurement TI2/2 -> RMS1/1, To Workspace4/1
  Measurement TI2/1 -> RMS2/1, To Workspace6/1
  RMS2/1 -> Display2/1
  Measurement TI3/1 -> RMS4/1
  RMS1/1 -> Display1/1
  Measurement TI3/2 -> RMS3/1
  RMS3/1 -> Display3/1
  RMS4/1 -> Display4/1
  Measurement TI1/2 -> RMS5/1, To Workspace7/1
  RMS5/1 -> Display5/1
  connections:
  Ze/LConn1 -- Measurement TI1/RConn3
  Measurement TI1/LConn3 -- TI/RConn3
  Ze/RConn1 -- Raterr(TI)/LConn1
  TC1/LConn3 -- Raterr(TI)3/RConn1
  FuseB3/LConn1 -- TC1/LConn2
  Raterr(TI)2/RConn1 -- TC/LConn3
  Raterr(TI)4/RConn1 -- Raterr(TI)1/RConn1 -- Raterr(TI)5/RConn1
  Raterr(TI)7/RConn1 -- Raterr(TI)6/RConn1 -- Raterr(TI)8/RConn1
  Raterr(TI)/RConn1 -- Modelo Linha Curtos/LConn3
  Three-Phase Series RLC Load/LConn2 -- TC1/RConn2
  Three-Phase Series RLC Load/LConn1 -- TC1/RConn1
  Three-Phase Series RLC Load/LConn3 -- TC1/RConn3
  Three-Phase Series RLC Load4/LConn1 -- TC/RConn1
  Three-Phase Series RLC Load4/LConn2 -- TC/RConn2
  Three-Phase Series RLC Load4/LConn3 -- TC/RConn3
  TI/LConn1 -- FuseA/LConn1
  FuseB/LConn1 -- TI/LConn2
  TI/LConn3 -- FuseC/LConn1
  FuseB1/LConn1 -- Measurement TI1/LConn2
  FuseA1/LConn1 -- Measurement TI1/LConn1
  TI/RConn1 -- FuseA1/RConn1
  FuseB1/RConn1 -- TI/RConn2
  FuseB2/LConn1 -- TC/LConn2
  TC/LConn1 -- FuseA2/LConn1
  FuseA3/LConn1 -- TC1/LConn1
  FuseB/RConn1 -- Measurement TI2/RConn2
  Measurement TI3/RConn3 -- TI1/LConn3
  Measurement TI2/LConn3 -- TI1/RConn3
  Measurement TI3/LConn2 -- Three-Phase Source/RConn2
  TI1/LConn1 -- Measurement TI3/RConn1
  FuseC/RConn1 -- Measurement TI2/RConn3
  FuseA/RConn1 -- Measurement TI2/RConn1
  TI1/RConn1 -- Measurement TI2/LConn1
  Measurement TI3/RConn2 -- TI1/LConn2
  Measurement TI3/LConn3 -- Three-Phase Source/RConn3
  TI1/RConn2 -- Measurement TI2/LConn2
  Measurement TI3/LConn1 -- Three-Phase Source/RConn1
  Measurement TI1/RConn1 -- Modelo Linha Curtos/LConn1
  Measurement TI1/RConn2 -- Modelo Linha Curtos/LConn2
  Modelo Linha Curtos/RConn3 -- Raterr(TI)2/LConn1 -- Raterr(TI)5/LConn1 -- Modelo Linha 2/LConn3
  Modelo Linha Curtos/RConn2 -- Raterr(TI)4/LConn1 -- FuseB2/RConn1 -- Modelo Linha 2/LConn2
  Modelo Linha Curtos/RConn1 -- Raterr(TI)1/LConn1 -- FuseA2/RConn1 -- Modelo Linha 2/LConn1
  Modelo Linha 2/RConn3 -- Raterr(TI)8/LConn1 -- Raterr(TI)3/LConn1
  FuseB3/RConn1 -- Raterr(TI)7/LConn1 -- Modelo Linha 2/RConn2
  Modelo Linha 2/RConn1 -- Raterr(TI)6/LConn1 -- FuseA3/RConn1
